simulink model "inputs_o"  (R2023a)
settings: Solver=VariableStepAuto  StartTime=0.0  StopTime=10.0  RelTol=1e-3
settings Model: Creator=u29w13  LastModifiedBy=u29w13

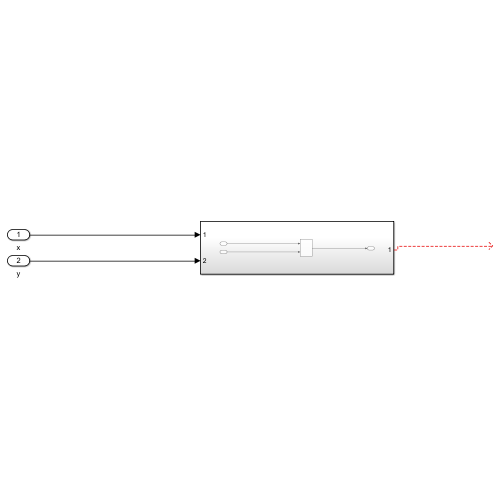
[thumbnail: Simulink's stored preview of the top-level diagram]
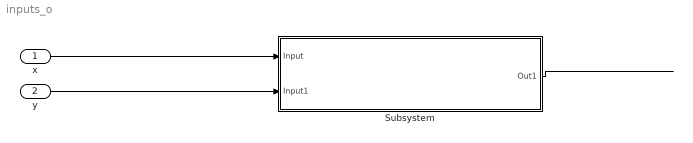
== system inputs_o ==
  x : Inport
  y : Inport  Port=2
  Subsystem : Subsystem
  wires:
  x/1 -> Subsystem/1(Input)
  Subsystem/1(Out1) -> ?
  y/1 -> Subsystem/2(Input1)

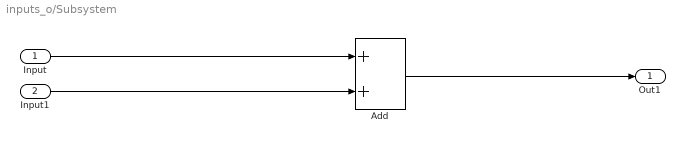
== system inputs_o/Subsystem ==
  Input : Inport
  Input1 : Inport  Port=2
  Add : Sum
  Out1 : Outport
  wires:
  Input/1 -> Add/1
  Input1/1 -> Add/2
  Add/1 -> Out1/1
